simulink model "turbofan"  (R2018a)
settings: Solver=VariableStepAuto  StartTime=0.0  StopTime=0.0  RelTol=1e-3
libraries: motorlib x7
settings Model: Creator=mairon  LastModifiedBy=mairon

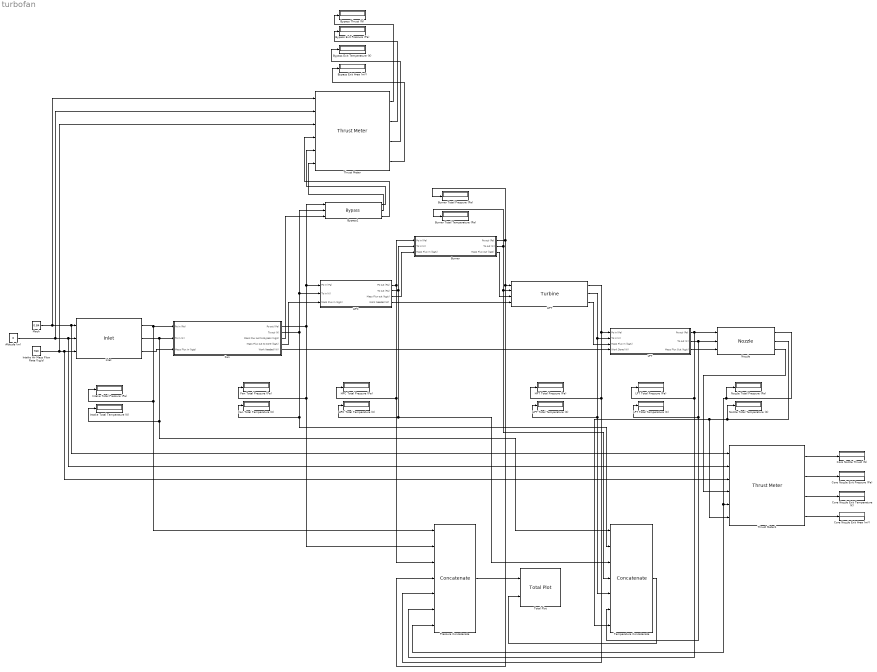
== system turbofan ==
  Altitude (m) : Constant  Value=0
  Burner : Subsystem  AncestorBlock=motorlib/Burner
  Burner Total Pressure (Pa) : Display
  Burner Total Temperature (Pa) : Display
  Bypass Exit Area (m²) : Display
  Bypass Exit Pressure (Pa) : Display
  Bypass Exit Temperature (K) : Display
  Bypass Thrust (N) : Display
  Bypass1 : motorlib/Bypass
      settings: SourceProductName=Aeronautic Motor
  Core Nozzle Exit Area (m²) : Display
  Core Nozzle Exit Pressure (Pa) : Display
  Core Nozzle Exit Temperature (K) : Display
  Core Nozzle Thrust (N) : Display
  Fan : Subsystem  AncestorBlock=motorlib/Fan
  Fan Total Pressure (Pa) : Display
  Fan Total Temperature (K) : Display
  HPC : Subsystem  AncestorBlock=motorlib/Compressor
  HPC Total Pressure (Pa) : Display
  HPC Total Temperature (K) : Display
  HPT : motorlib/Turbine
      settings: SourceProductName=Aeronautic Motor
  HPT Total Pressure (Pa) : Display
  HPT Total Temperature (K) : Display
  Inlet : motorlib/Inlet
      settings: SourceProductName=Aeronautic Motor
  Intake Air Mass Flow Rate (kg/s) : Constant  Value=780
  Intake Total Pressure (Pa) : Display
  Intake Total Temperature (K) : Display
  LPT : Subsystem  AncestorBlock=motorlib/Turbine
  LPT Total Pressure (Pa) : Display
  LPT Total Temperature (K) : Display
  Mach : Constant  Value=0.84
  Nozzle : motorlib/Nozzle
      settings: SourceProductName=Aeronautic Motor
  Nozzle Total Pressure (Pa) : Display
  Nozzle Total Temperature (K) : Display
  Pressure Concatenate : Concatenate  NumInputs=7
  Temperature Concatenate : Concatenate  NumInputs=7
  Thrust Meter : motorlib/Thrust Meter
      settings: SourceProductName=Aeronautic Motor
  Thrust Meter1 : motorlib/Thrust Meter
      settings: SourceProductName=Aeronautic Motor
  Total Plot : motorlib/Total Plot
      settings: SourceProductName=Stateflow  SourceProductBaseCode=SF
  wires:
  Inlet/1 -> Fan/1(Po in (Pa)), Pressure Concatenate/1, Intake Total Pressure (Pa)/1
  Inlet/2 -> Temperature Concatenate/1, Intake Total Temperature (K)/1, Fan/2(To in (K))
  HPC/4(Work Needed (W)) -> HPT/4
  HPC/1(Po out (Pa)) -> Burner/1(Po in (Pa)), Pressure Concatenate/3, HPC Total Pressure (Pa)/1
  HPC/2(To out (Pa)) -> Burner/2(To in (K)), Temperature Concatenate/3, HPC Total Temperature (K)/1
  HPC/3(Mass Flux out (kg/s)) -> Burner/3(Mass Flux in (kg/s))
  Burner/1(Po out (Pa)) -> HPT/1, Pressure Concatenate/4, Burner Total Pressure (Pa)/1
  Burner/2(To out (K)) -> Temperature Concatenate/4, HPT/2, Burner Total Temperature (Pa)/1
  Burner/3(Mass Flux out (kg/s)) -> HPT/3
  HPT/1 -> LPT/1(Po in (Pa)), Pressure Concatenate/5, HPT Total Pressure (Pa)/1
  HPT/2 -> LPT/2(To in (K)), Temperature Concatenate/5, HPT Total Temperature (K)/1
  HPT/3 -> LPT/3(Mass Flux in (kg/s))
  LPT/1(Po out (Pa)) -> Nozzle/1, Pressure Concatenate/6, LPT Total Pressure (Pa)/1
  LPT/2(To out (K)) -> Nozzle/2, Temperature Concatenate/6, LPT Total Temperature (K)/1
  LPT/3(Mass Flux Out (kg/s)) -> Nozzle/3
  Altitude (m)/1 -> Thrust Meter/2, Inlet/2, Thrust Meter1/2
  Mach/1 -> Thrust Meter/1, Inlet/1, Thrust Meter1/1
  Intake Air Mass Flow Rate (kg/s)/1 -> Thrust Meter/3, Inlet/3, Thrust Meter1/3
  Fan/1(Po out (Pa)) -> Bypass1/1, HPC/1(Po in (Pa)), Pressure Concatenate/2, Fan Total Pressure (Pa)/1
  Fan/2(To out (K)) -> Bypass1/2, HPC/2(To in (K)), Temperature Concatenate/2, Fan Total Temperature (K)/1
  Fan/4(Mass Flux out to Core (kg/s)) -> HPC/3(Mass Flux in (kg/s))
  Fan/5(Work Needed (W)) -> LPT/4(Work Done (W))
  Nozzle/1 -> Pressure Concatenate/7, Thrust Meter1/5, Nozzle Total Pressure (Pa)/1
  Nozzle/2 -> Temperature Concatenate/7, Thrust Meter1/6, Nozzle Total Temperature (K)/1
  Inlet/3 -> Fan/3(Mass Flux in (kg/s))
  Fan/3(Mass Flux out to Bypass (kg/s)) -> Bypass1/3
  Bypass1/1 -> Thrust Meter/5
  Bypass1/2 -> Thrust Meter/6
  Bypass1/3 -> Thrust Meter/4
  Thrust Meter/1 -> Bypass Thrust (N)/1
  Thrust Meter/2 -> Bypass Exit Pressure (Pa)/1
  Thrust Meter/3 -> Bypass Exit Temperature (K)/1
  Thrust Meter/4 -> Bypass Exit Area (m²)/1
  Nozzle/3 -> Thrust Meter1/4
  Thrust Meter1/1 -> Core Nozzle Thrust (N)/1
  Thrust Meter1/2 -> Core Nozzle Exit Pressure (Pa)/1
  Thrust Meter1/3 -> Core Nozzle Exit Temperature (K)/1
  Thrust Meter1/4 -> Core Nozzle Exit Area (m²)/1
  Pressure Concatenate/1 -> Total Plot/1
  Temperature Concatenate/1 -> Total Plot/2

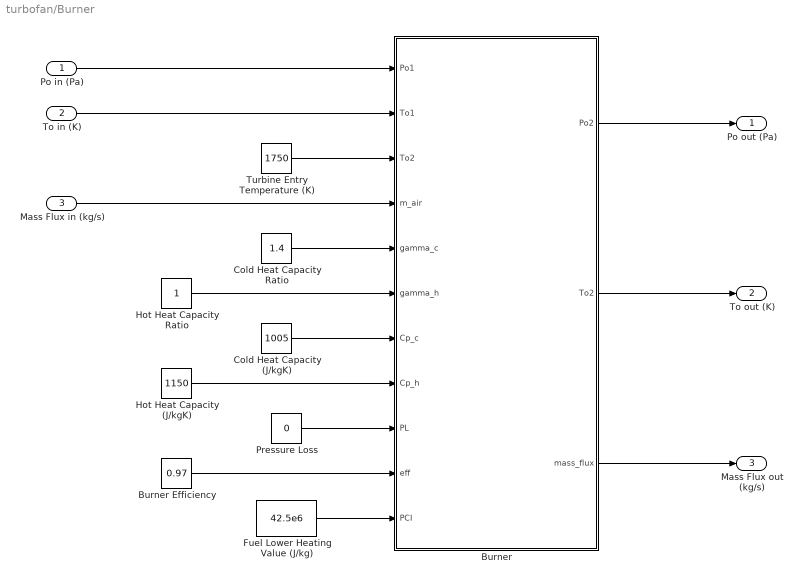
== system turbofan/Burner ==
  Po in (Pa) : Inport
  To in (K) : Inport  Port=2
  Mass Flux in (kg/s) : Inport  Port=3
  Burner : MATLAB Function  TreatAsAtomicUnit=on
  Burner Efficiency : Constant  Value=0.97
  Cold Heat Capacity (J/kgK) : Constant  Value=1005
  Cold Heat Capacity Ratio : Constant  Value=1.4
  Fuel Lower Heating Value (J/kg) : Constant  Value=42.5e6
  Hot Heat Capacity (J/kgK) : Constant  Value=1150
  Hot Heat Capacity Ratio : Constant
  Pressure Loss : Constant  Value=0
  Turbine Entry Temperature (K) : Constant  Value=1750
  Po out (Pa) : Outport
  To out (K) : Outport  Port=2
  Mass Flux out (kg/s) : Outport  Port=3
  wires:
  Hot Heat Capacity Ratio/1 -> Burner/6(gamma_h)
  Burner Efficiency/1 -> Burner/10(eff)
  Burner/1(Po2) -> Po out (Pa)/1
  Mass Flux in (kg/s)/1 -> Burner/4(m_air)
  Cold Heat Capacity Ratio/1 -> Burner/5(gamma_c)
  Fuel Lower Heating Value (J/kg)/1 -> Burner/11(PCI)
  Burner/3(mass_flux) -> Mass Flux out (kg/s)/1
  To in (K)/1 -> Burner/2(To1)
  Hot Heat Capacity (J/kgK)/1 -> Burner/8(Cp_h)
  Turbine Entry Temperature (K)/1 -> Burner/3("To2 ")
  Burner/2(To2) -> To out (K)/1
  Po in (Pa)/1 -> Burner/1(Po1)
  Pressure Loss/1 -> Burner/9(PL)
  Cold Heat Capacity (J/kgK)/1 -> Burner/7(Cp_c)

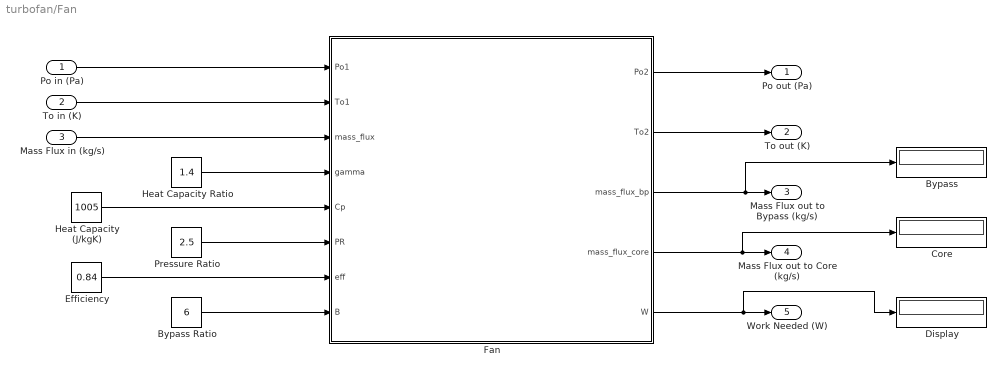
== system turbofan/Fan ==
  Po in (Pa) : Inport
  To in (K) : Inport  Port=2
  Mass Flux in (kg/s) : Inport  Port=3
  Bypass : Display
  Bypass Ratio : Constant  Value=6
  Core : Display
  Display : Display
  Efficiency : Constant  Value=0.84
  Fan : MATLAB Function  TreatAsAtomicUnit=on
  Heat Capacity (J/kgK) : Constant  Value=1005
  Heat Capacity Ratio : Constant  Value=1.4
  Pressure Ratio : Constant  Value=2.5
  Po out (Pa) : Outport
  To out (K) : Outport  Port=2
  Mass Flux out to Bypass (kg/s) : Outport  Port=3
  Mass Flux out to Core (kg/s) : Outport  Port=4
  Work Needed (W) : Outport  Port=5
  wires:
  Pressure Ratio/1 -> Fan/6(PR)
  Mass Flux in (kg/s)/1 -> Fan/3(mass_flux)
  Bypass Ratio/1 -> Fan/8(B)
  To in (K)/1 -> Fan/2(To1)
  Heat Capacity Ratio/1 -> Fan/4(gamma)
  Efficiency/1 -> Fan/7(eff)
  Fan/3(mass_flux_bp) -> Bypass/1, Mass Flux out to Bypass (kg/s)/1
  Fan/5(W) -> Display/1, Work Needed (W)/1
  Fan/4(mass_flux_core) -> Core/1, Mass Flux out to Core (kg/s)/1
  Heat Capacity (J/kgK)/1 -> Fan/5(Cp)
  Fan/2(To2) -> To out (K)/1
  Po in (Pa)/1 -> Fan/1(Po1)
  Fan/1(Po2) -> Po out (Pa)/1

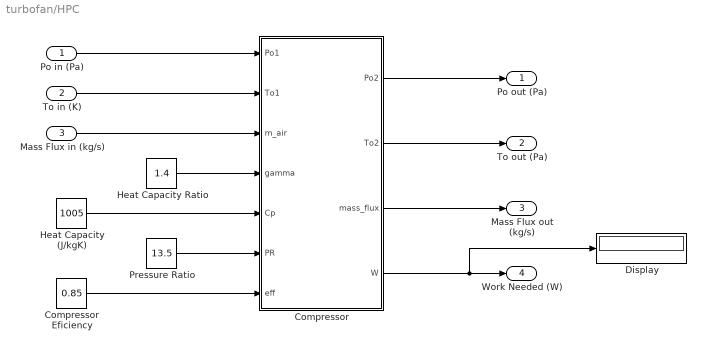
== system turbofan/HPC ==
  Po in (Pa) : Inport
  To in (K) : Inport  Port=2
  Mass Flux in (kg/s) : Inport  Port=3
  Compressor : MATLAB Function  TreatAsAtomicUnit=on
  Compressor Eficiency : Constant  Value=0.85
  Display : Display
  Heat Capacity (J/kgK) : Constant  Value=1005
  Heat Capacity Ratio : Constant  Value=1.4
  Pressure Ratio : Constant  Value=13.5
  Po out (Pa) : Outport
  To out (Pa) : Outport  Port=2
  Mass Flux out (kg/s) : Outport  Port=3
  Work Needed (W) : Outport  Port=4
  wires:
  Compressor Eficiency/1 -> Compressor/7(eff)
  Pressure Ratio/1 -> Compressor/6(PR)
  Heat Capacity (J/kgK)/1 -> Compressor/5(Cp)
  Heat Capacity Ratio/1 -> Compressor/4(gamma)
  Compressor/3(mass_flux) -> Mass Flux out (kg/s)/1
  To in (K)/1 -> Compressor/2(To1)
  Compressor/1(Po2) -> Po out (Pa)/1
  Po in (Pa)/1 -> Compressor/1(Po1)
  Compressor/2(To2) -> To out (Pa)/1
  Compressor/4(W) -> Display/1, Work Needed (W)/1
  Mass Flux in (kg/s)/1 -> Compressor/3(m_air)

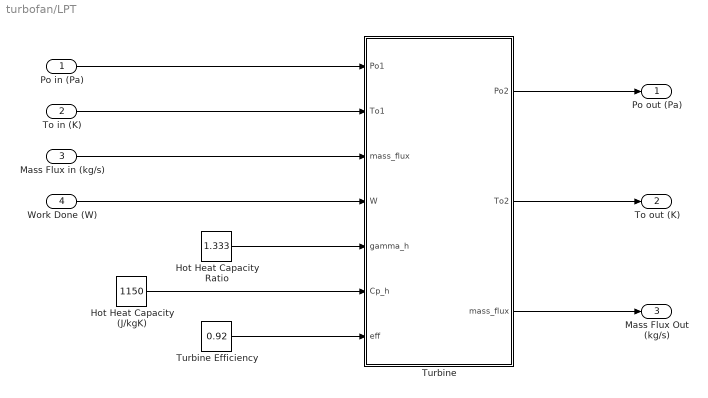
== system turbofan/LPT ==
  Po in (Pa) : Inport
  To in (K) : Inport  Port=2
  Mass Flux in (kg/s) : Inport  Port=3
  Work Done (W) : Inport  Port=4
  Hot Heat Capacity (J/kgK) : Constant  Value=1150
  Hot Heat Capacity Ratio : Constant  Value=1.333
  Turbine : MATLAB Function  TreatAsAtomicUnit=on
  Turbine Efficiency : Constant  Value=0.92
  Po out (Pa) : Outport
  To out (K) : Outport  Port=2
  Mass Flux Out (kg/s) : Outport  Port=3
  wires:
  Mass Flux in (kg/s)/1 -> Turbine/3("mass_flux ")
  Po in (Pa)/1 -> Turbine/1(Po1)
  Turbine Efficiency/1 -> Turbine/7(eff)
  Turbine/3(mass_flux) -> Mass Flux Out (kg/s)/1
  Hot Heat Capacity Ratio/1 -> Turbine/5(gamma_h)
  Hot Heat Capacity (J/kgK)/1 -> Turbine/6(Cp_h)
  Turbine/1(Po2) -> Po out (Pa)/1
  Work Done (W)/1 -> Turbine/4(W)
  To in (K)/1 -> Turbine/2(To1)
  Turbine/2(To2) -> To out (K)/1

== matlab function turbofan/HPC/Compressor ==
  data: Po2 output; To2 output; mass_flux output; Po1 input; To1 input; m_air input; W output; gamma input; Cp input; PR input; eff input
function [Po2,To2,mass_flux,W] = Compressor(Po1,To1,m_air,gamma,Cp,PR,eff)
    Po2 = PR*Po1;   % total pressure out
    To2s = PR^((gamma-1)/gamma) * To1;  % total isentropic temperature out
    To2 = (To2s-To1)/eff + To1; % total temperature out
    
    mass_flux = m_air; % mass flux out
   
    W=m_air*Cp*(To1-To2); % work used by the compressor

== matlab function turbofan/Burner/Burner ==
  data: Po1 input; Po2 output; To2 output; To1 input; To2 input; mass_flux output; m_air input; gamma_c input; gamma_h input; Cp_c input; Cp_h input; PL input; eff input; PCI input
function [Po2,To2,mass_flux] = Burner(Po1,To1,To2,m_air,gamma_c,gamma_h,Cp_c,Cp_h,PL,eff,PCI)
    PR = 1 - PL;    % pressure ratio   
    Po2 = PR*Po1;
    
    f=(Cp_h*To2 - Cp_c*To1)/(eff*PCI + Cp_h*To2);
    
    m_f = m_air*f;
    mass_flux = m_air + m_f;

== matlab function turbofan/LPT/Turbine ==
  data: Po1 input; To1 input; mass_flux input; W input; Po2 output; To2 output; gamma_h input; Cp_h input; eff input; mass_flux output
function [Po2,To2,mass_flux]  = Turbine(Po1,To1,mass_flux,W,gamma_h,Cp_h,eff)   
    To2 = W/(Cp_h*mass_flux) + To1; % real total temperature
    To2s = (To2-To1)/eff + To1; % isentropic total temperature
    
    PR = (To2s/To1)^(gamma_h/(gamma_h-1));   % pressure ratio
    Po2 = PR*Po1;   % total pressure

== matlab function turbofan/Fan/Fan ==
  data: Po1 input; To1 input; mass_flux input; gamma input; Cp input; PR input; eff input; B input; Po2 output; To2 output; mass_flux_bp output; mass_flux_core output; W output
function [Po2,To2,mass_flux_bp,mass_flux_core,W] = Fan(Po1,To1,mass_flux,gamma,Cp,PR,eff,B)
    Po2 = PR*Po1;   % total pressure out
    To2s = PR^((gamma-1)/gamma) * To1;  % total isentropic temperature out
    To2 = (To2s-To1)/eff + To1; % total temperature out
    
    W=mass_flux*Cp*(To1-To2); % work used by the compressor
    
    mass_flux_core = mass_flux/(1+B); % mass flux out to the core
    mass_flux_bp = mass_flux - mass_flux_core; % mass flux out to bypass
